simulink library "ModG_Neumatico"  (R2018a)
settings: Solver=VariableStepAuto  StartTime=0.0  StopTime=10.0  RelTol=1e-3
undefined symbols (not defined in the file): Calfa, GR, low_v, mu_s, mux, muy, Rg, sc
libraries: ModG_Transformaciones x8, $bdroot x2
settings Model: Creator=Lisandro Cocca  LastModifiedBy=Lisandro Cocca

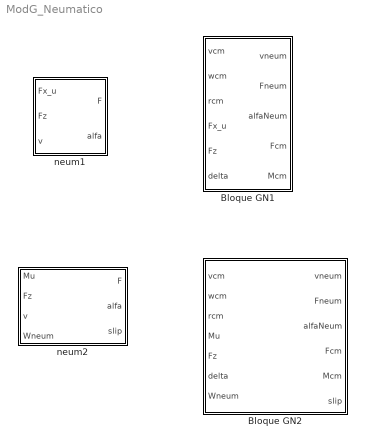
== system ModG_Neumatico ==
  Bloque GN1 : Subsystem  mask{mux=1, muy=1, Calfa=1}
      mask prompts: mux "Coeficiente de roce longitudinal max 'mux' = Fxmax/Fz"; muy "Coeficiente de roce longitudinal max 'muy' = Fymax/Fz"; Calfa "Coeficiente lineal de Fy 'Calfa'"
  Bloque GN2 : Subsystem  mask{muy=1, Calfa=1, low_v=0.1, mu_s=1, sc=0.75}
      mask prompts: muy "Coeficiente de roce longitudinal max 'muy' = Fymax/Fz"; Calfa "Coeficiente lineal de Fy 'Calfa'"; low_v "Velocidad minima p/doblar 'low_v'"; mu_s "Sliding value mux 'mu_s'"; sc "Slip critico"
  neum1 : Subsystem
  neum2 : Subsystem

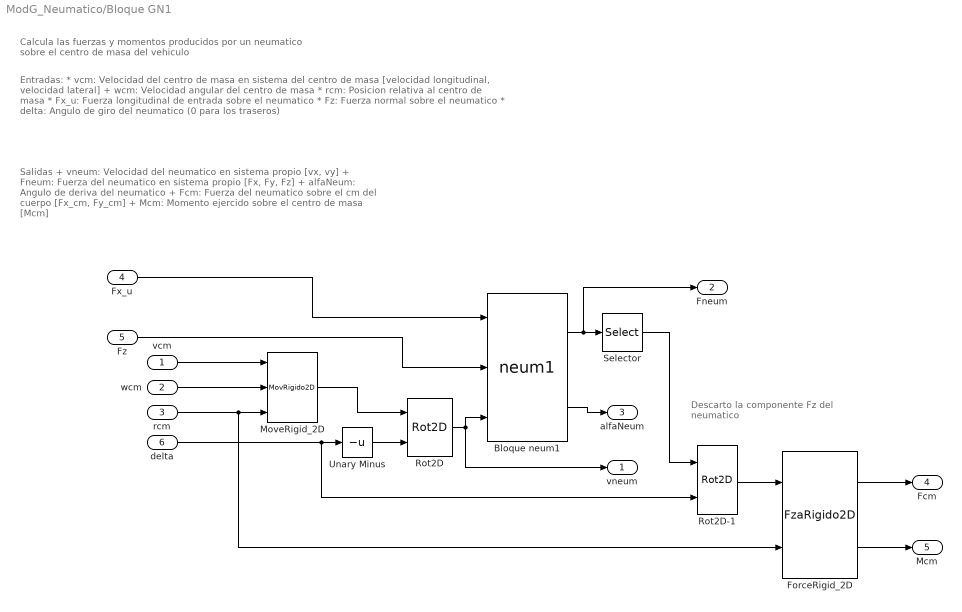
== system ModG_Neumatico/Bloque GN1 ==
  note: Calcula las fuerzas y momentos producidos por un neumatico
      | sobre el centro de masa del vehiculo
  note: Entradas:
      | 	* vcm: Velocidad del centro de masa en sistema del centro de masa [velocidad longitudinal, velocidad lateral]
      | 	+ wcm: Velocidad angular del centro de masa
      | 	* rcm: Posicion relativa al centro de masa
      | 	* Fx_u: Fuerza longitudinal de entrada sobre el neumatico
      | 	* Fz: Fuerza normal sobre el neumatico
      | 	* delta: Angulo de giro del neumatico (0 para los traseros)
  note: Salidas
      | 	+ vneum: Velocidad del neumatico en sistema propio [vx, vy]
      | 	+ Fneum: Fuerza del neumatico en sistema propio [Fx, Fy, Fz]
      | 	+ alfaNeum: Angulo de deriva del neumatico
      | 	+ Fcm: Fuerza del neumatico sobre el cm del cuerpo [Fx_cm, Fy_cm]
      | 	+ Mcm: Momento ejercido sobre el centro de masa [Mcm]
  note: Descarto la componente
      | Fz del neumatico
  vcm : Inport
  wcm : Inport  Port=2
  rcm : Inport  Port=3
  Fx_u : Inport  Port=4
  Fz : Inport  Port=5
  delta : Inport  Port=6
  Bloque neum1 : $bdroot/neum1
  ForceRigid_2D : ModG_Transformaciones/FzaRigido2D
  MoveRigid_2D : ModG_Transformaciones/MovRigido2D
  Rot2D : ModG_Transformaciones/Rot2D
  Rot2D-1 : ModG_Transformaciones/Rot2D
  Selector : Selector  InputPortWidth=3  IndexOptions=Index vector (dialog)  Indices=[1 2]  OutputSizes=1
  Unary Minus : UnaryMinus
  vneum : Outport
  Fneum : Outport  Port=2
  alfaNeum : Outport  Port=3
  Fcm : Outport  Port=4
  Mcm : Outport  Port=5
  wires:
  ForceRigid_2D/1 -> Fcm/1
  wcm/1 -> MoveRigid_2D/2
  rcm/1 -> ForceRigid_2D/2, MoveRigid_2D/3
  ForceRigid_2D/2 -> Mcm/1
  Rot2D/1 -> vneum/1, Bloque neum1/3
  Selector/1 -> Rot2D-1/1
  Fx_u/1 -> Bloque neum1/1
  MoveRigid_2D/1 -> Rot2D/1
  vcm/1 -> MoveRigid_2D/1
  Rot2D-1/1 -> ForceRigid_2D/1
  Bloque neum1/1 -> Fneum/1, Selector/1
  delta/1 -> Rot2D-1/2, Unary Minus/1
  Unary Minus/1 -> Rot2D/2
  Fz/1 -> Bloque neum1/2
  Bloque neum1/2 -> alfaNeum/1

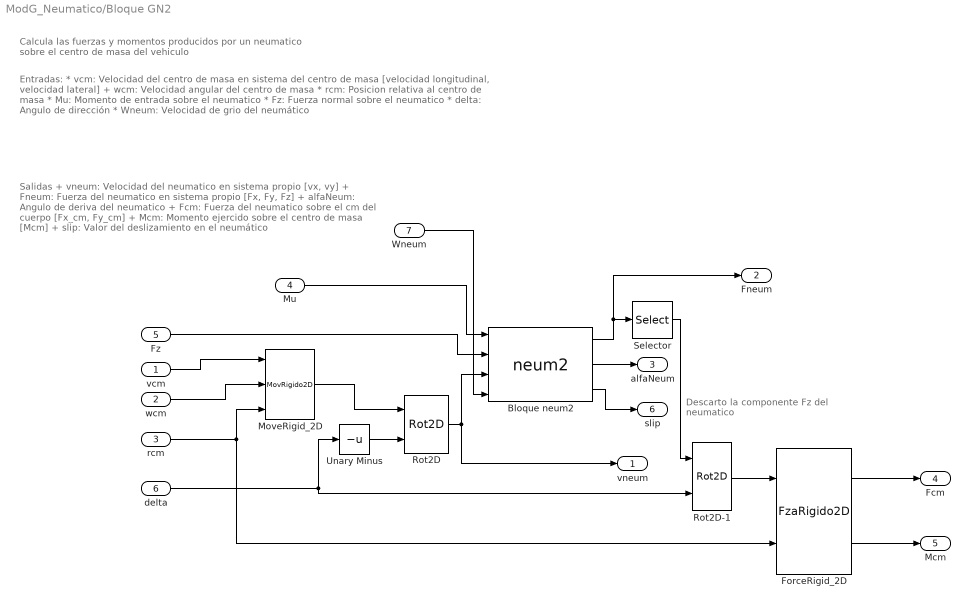
== system ModG_Neumatico/Bloque GN2 ==
  note: Descarto la componente
      | Fz del neumatico
  note: Calcula las fuerzas y momentos producidos por un neumatico
      | sobre el centro de masa del vehiculo
  note: Entradas:
      | 	* vcm: Velocidad del centro de masa en sistema del centro de masa [velocidad longitudinal, velocidad lateral]
      | 	+ wcm: Velocidad angular del centro de masa
      | 	* rcm: Posicion relativa al centro de masa
      | 	* Mu: Momento de entrada sobre el neumatico
      | 	* Fz: Fuerza normal sobre el neumatico
      | 	* delta: Angulo de dirección
      | 	* Wneum: Velocidad de grio del neumático
  note: Salidas
      | 	+ vneum: Velocidad del neumatico en sistema propio [vx, vy]
      | 	+ Fneum: Fuerza del neumatico en sistema propio [Fx, Fy, Fz]
      | 	+ alfaNeum: Angulo de deriva del neumatico
      | 	+ Fcm: Fuerza del neumatico sobre el cm del cuerpo [Fx_cm, Fy_cm]
      | 	+ Mcm: Momento ejercido sobre el centro de masa [Mcm]
      | 	+ slip: Valor del deslizamiento en el neumático
  vcm : Inport
  wcm : Inport  Port=2
  rcm : Inport  Port=3
  Mu : Inport  Port=4
  Fz : Inport  Port=5
  delta : Inport  Port=6
  Wneum : Inport  Port=7
  Bloque neum2 : $bdroot/neum2
  ForceRigid_2D : ModG_Transformaciones/FzaRigido2D
  MoveRigid_2D : ModG_Transformaciones/MovRigido2D
  Rot2D : ModG_Transformaciones/Rot2D
  Rot2D-1 : ModG_Transformaciones/Rot2D
  Selector : Selector  InputPortWidth=3  IndexOptions=Index vector (dialog)  Indices=[1 2]  OutputSizes=1
  Unary Minus : UnaryMinus
  vneum : Outport
  Fneum : Outport  Port=2
  alfaNeum : Outport  Port=3
  Fcm : Outport  Port=4
  Mcm : Outport  Port=5
  slip : Outport  Port=6
  wires:
  Bloque neum2/1 -> Fneum/1, Selector/1
  delta/1 -> Unary Minus/1, Rot2D-1/2
  ForceRigid_2D/1 -> Fcm/1
  ForceRigid_2D/2 -> Mcm/1
  Wneum/1 -> Bloque neum2/4
  Rot2D-1/1 -> ForceRigid_2D/1
  Bloque neum2/2 -> alfaNeum/1
  Mu/1 -> Bloque neum2/1
  Selector/1 -> Rot2D-1/1
  wcm/1 -> MoveRigid_2D/2
  rcm/1 -> MoveRigid_2D/3, ForceRigid_2D/2
  Unary Minus/1 -> Rot2D/2
  vcm/1 -> MoveRigid_2D/1
  Rot2D/1 -> vneum/1, Bloque neum2/3
  Fz/1 -> Bloque neum2/2
  MoveRigid_2D/1 -> Rot2D/1
  Bloque neum2/3 -> slip/1

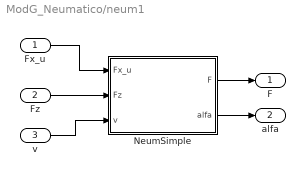
== system ModG_Neumatico/neum1 ==
  Fx_u : Inport  PortDimensions=1
  Fz : Inport  Port=2  PortDimensions=1
  v : Inport  Port=3  PortDimensions=2
  NeumSimple : MATLAB Function  TreatAsAtomicUnit=on
  F : Outport  PortDimensions=3
  alfa : Outport  Port=2  PortDimensions=1
  wires:
  Fz/1 -> NeumSimple/2(Fz)
  NeumSimple/1(F) -> F/1
  Fx_u/1 -> NeumSimple/1(Fx_u)
  v/1 -> NeumSimple/3(v)
  NeumSimple/2(alfa) -> alfa/1

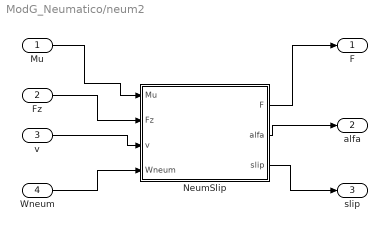
== system ModG_Neumatico/neum2 ==
  Mu : Inport  PortDimensions=1
  Fz : Inport  Port=2  PortDimensions=1
  v : Inport  Port=3  PortDimensions=2
  Wneum : Inport  Port=4  PortDimensions=1
  NeumSlip : MATLAB Function  TreatAsAtomicUnit=on
  F : Outport  PortDimensions=3
  alfa : Outport  Port=2  PortDimensions=1
  slip : Outport  Port=3  PortDimensions=1
  wires:
  Mu/1 -> NeumSlip/1(Mu)
  NeumSlip/2(alfa) -> alfa/1
  Fz/1 -> NeumSlip/2(Fz)
  v/1 -> NeumSlip/3(v)
  NeumSlip/1(F) -> F/1
  Wneum/1 -> NeumSlip/4(Wneum)
  NeumSlip/3(slip) -> slip/1

== matlab function ModG_Neumatico/neum2/NeumSlip ==
  data muy settings: description=Coeficiente de roce longitudinal max 'muy' = Fymax/Fz
  data Calfa settings: description=Coeficiente lineal de Fy 'Calfa'
  data: Mu input; F output size=3; Fz input; v input; Wneum input; muy parameter; Calfa parameter; alfa output; low_v parameter; slip output; Rg parameter; sc parameter; GR parameter; mu_s parameter
function [F, alfa, slip]  = neumSlip(Mu, Fz, v, Wneum, muy, Calfa, low_v, Rg, sc, GR, mu_s)
% Modelo de neumático simple (Sin inercia en la rueda)
% En el sentido longitudinal (x) limita la fuerza de entrada Fx_u si supera
% un cierto valor.
% En el sentido lateral (y) es proporcional al angulo de deriva (alfa)

% Salidas:
%   F: vector fuerza [Fx, Fy, Fz] del neumatico
%   alfa: Angulo de deriva del neumatico
%   slip: Es el deslizamiento entre la velocidad longitudinal y lateral del
%   neumatico

% Entradas:
%   Fx_u: Es la fuerza de entrada (Aplicada directamente en el parche de
%   contacto
%   Fz: Es la fuerza normal sobre el neumático
%   v: Es el vector velocidad en coordenadas de neumatico

%% Longitudinal Force

% Calculo del slip con correcion a baja velocidad
if abs(v(1)) > low_v
    slip = (Rg * Wneum / (v(1))) - 1;
else
    slip = 1*(Rg*Wneum);
end

% Definicion del mux con la función atan
mux = mu_s * tanh(slip/sc);
% Ver el tema de la sigmoide
Fx = mux * Fz;

%% Lateral Force
alfa = 0.0;
% A menos de esta velocidad no dobla el auto
if abs(v(1)) > low_v
    alfa = atan(v(2) / v(1));
end

% Ver el tema de la sigmoide
Fy = -Fz*Calfa*tanh(alfa);

F = [Fx, Fy, Fz]';

== matlab function ModG_Neumatico/neum1/NeumSimple ==
  data mux settings: description=Coeficiente de roce longitudinal max 'mux' = Fxmax/Fz
  data muy settings: description=Coeficiente de roce longitudinal max 'muy' = Fymax/Fz
  data Calfa settings: description=Coeficiente lineal de Fy 'Calfa'
  data: Fx_u input; F output; Fz input; v input; mux parameter; muy parameter; Calfa parameter; alfa output
function [F, alfa]  = neumSimple(Fx_u, Fz, v, mux, muy, Calfa)
% Modelo de neumático simple (Sin inercia en la rueda)
% En el sentido longitudinal (x) limita la fuerza de entrada Fx_u si supera
% un cierto valor.
% En el sentido lateral (y) es proporcional al angulo de deriva (alfa)
% Salidas:
%   F: vector fuerza [Fx, Fy, Fz] del neumatico
%   alfa: Angulo de deriva del neumatico
% Entradas:
%   Fx_u: Es la fuerza de entrada (Aplicada directamente en el parche de
%   contacto
%   Fz: Es la fuerza normal sobre el neumático
%   v: Es el vector velocidad en coordenadas de neumatico

if abs(Fx_u) <= mux * Fz
    Fx = Fx_u;
else
    Fx = sign(Fx_u)*mux*Fz;
end
if abs(v(1)) < 0.1 % A menos de esta velocidad no dobla el auto
    v(1) = 1;
    v(2) = 0;
    alfa = 0;
else
    alfa = atan(v(2) / v(1));
end
Fy_u = -Calfa*alfa*Fz;
if abs(Fy_u) < muy*Fz
    Fy = Fy_u;
else
    Fy = sign(Fy_u)*muy*Fz;
end

F = [Fx, Fy, Fz]';
